simulink model "Demo_Shore"  (R2014a)
settings: Solver=FixedStepDiscrete  SolverMode=SingleTasking  StartTime=0.0  StopTime=inf  FixedStep=0.01  RelTol=1e-3
PostLoadFcn:
  | h_RPStest = RPStest;
model workspace (MAT data in the model file):
  gtest = 0
undefined symbols (not defined in the file or in its folder): avert, avert_gaze_dirs_chance, avert_gaze_duration_factor, avert_head_frequency_factor, avert_head_speed, BML, BML1, BML2, bmlsL, bmlsM, bodyBusyFlag, clock, emotion_amount_factor, faceBusyFlag, fileID, GAZE_WIN, gazing, mutual_gaze_duration_factor, P, pose_chanc_factor, pose_chance_factor, pose_change_flag, pose_frequency_factor, pose_lean, pose_lean_flag, pose_selfAdaptor_chance_factor, pose_speed, pr, serial, STATE_BEFORE, STATE_GO, STATE_OVER, STATE_READY, Stateflow
libraries: simulink x23, instrumentlib x6, lib_affectiveChar_behavior x3, realtime_pacer_lib x2, lib_affectiveChar_input x1
(part 5 of 7)

== stateflow chart Demo_Shore/CharacterControl/personalSpace_Controller ==
  state stateInit
    entry: gameState=14;
    TOO_CLOSE=1;TOO_FAR=2;NEUTRAL=0;
    farBuffer=0;closeBuffer=0;neutralBuffer=0;position=1;
    n=encStr2Arr(' ');bmlsM=[n n n n n];newBmlsM=[n n n n n];
    bmlsL=[n n n n n];newBmlsL=[n n n n n];
  note: Problem:
      | Sometimes locomotion BML is sent (visible in the vhmsgYarpRelais) but it is not running. Also smartbody shows duplicate msg id error. It seems that when too many BMLs are sent to smartbody some of them have same IDs.
  state wait
  note: if avert not 1
  state gazeSurprized
    entry: [P,BMLM]=walkInvadingTable(5) ;
    closeBuffer=closeBuffer+1;
    newBmlsM=insertQueue(bmlsM,BMLM);
    bmlsM=newBmlsM;
  state doIt3Times
    entry: position=2;
    closeBuffer=0;
  note: User is too close!
  state headNeuralGazeCamera
    entry: [P,BMLM]=walkInvadingTable(4) ;
    newBmlsM=insertQueue(bmlsM,BMLM);
    bmlsM=newBmlsM;
  state stateWalkBack
    entry:  [P,BMLM]=walkInvadingTable(2);
    newBmlsM=insertQueue(bmlsM,BMLM);  bmlsM=newBmlsM;
    closeBuffer=closeBuffer+1;
  state browUp
    entry: [P,BMLM]=walkInvadingTable(8) ;
    neutralBuffer=neutralBuffer+1;
    newBmlsM=insertQueue(bmlsM,BMLM);
    bmlsM=newBmlsM;
  state doIt3Times1
    entry: position=1;
    neutralBuffer=0;
  note: EXE ORDER IMPORTANT
  state checkUserCoord
  note: correct: [zChange==1]{position=0;}
  state idle
    entry: [P,BMLM]=walkInvadingTable(1);
    newBmlsM=insertQueue(bmlsM,BMLM);
    bmlsM=newBmlsM;
    neutralBuffer=neutralBuffer+1;
  note: User is in the middle!
  state wait2
  state leanFW
    entry: [P,BMLM]=walkInvadingTable(6) ;
    farBuffer=farBuffer+1;
    newBmlsM=insertQueue(bmlsM,BMLM);
    bmlsM=newBmlsM;
  state doIt3Times2
    entry: position=3;
    farBuffer=0;
  note: Problem:
      | We dont know where smatbody is standing (z pos). If smartbody does not run the locomotion BML sent for any reason (too many BMLs), we want to send locomodation BML again after a while to make sure the personal space is correct. On the other hand, we dont want the module to keep sending move bmls.
  state walkFW
    entry:  [P,BMLM]=walkInvadingTable(3) ;
    newBmlsM=insertQueue(bmlsM,BMLM);  bmlsM=newBmlsM;
    farBuffer=farBuffer+1;
  note: User is too far!
  state leanNeutral
    entry:  [P,BMLM]=walkInvadingTable(7) ;
    newBmlsM=insertQueue(bmlsM,BMLM); bmlsM=newBmlsM;
  (default) -> stateInit
  stateInit -> (junction 2)
  wait -> (junction 2)
  (junction 2) -> headNeuralGazeCamera [order 1] : [avert==1]
  (junction 2) -> checkUserCoord [order 2]
  idle -> wait [order 2] : after(5,secs)
  walkFW -> wait [order 2] : after(5,secs)
  stateWalkBack -> wait [order 2] : after(5,secs)
  doIt3Times1 -> wait : after(5,secs)
  doIt3Times2 -> wait : after(5,secs)
  doIt3Times -> wait : after(5,secs)
  checkUserCoord -> (junction 89) [order 3] : [[distance==TOO_CLOSE]&[position~=2]]
  (junction 89) -> gazeSurprized [order 2] : [closeBuffer<2]
  (junction 89) -> stateWalkBack [order 1] : [closeBuffer>=2]
  stateWalkBack -> doIt3Times [order 1] : [closeBuffer==5]
  gazeSurprized -> checkUserCoord
  headNeuralGazeCamera -> checkUserCoord
  checkUserCoord -> (junction 92) [order 2] : [[distance==NEUTRAL]&[position~=1]]
  (junction 92) -> browUp [order 1] : [neutralBuffer<2]
  wait2 -> checkUserCoord [order 1] : [zChange==1]{position=0;}
  idle -> doIt3Times1 [order 1] : [neutralBuffer==5]
  browUp -> checkUserCoord
  (junction 92) -> idle [order 2] : [neutralBuffer>=2]
  wait2 -> checkUserCoord [order 2] : [zChange~=1]
  checkUserCoord -> wait2 [order 4] : after(20,secs)
  checkUserCoord -> (junction 87) [order 1] : [[distance==TOO_FAR]&[position~=3]]
  leanFW -> checkUserCoord
  (junction 87) -> leanFW [order 2] : [farBuffer<2]
  walkFW -> doIt3Times2 [order 1] : [farBuffer==5]
  (junction 87) -> leanNeutral [order 1] : [farBuffer>=2]
  leanNeutral -> walkFW : after(2,secs)
  data: bmls function_input double size=[1000,5]; myBML function_input double size=[1000,1]; newBmls function_output double size=[1000,5]; p function_output double size=1; bmlID function_input double size=1; poseBML function_output double size=[1000,1]; bmls function_input double size=[1000,5]; myBML function_input double size=[1000,1]; newBmls function_output double size=[1000,5]; gameState output double size=1; STATE_READY data_store_memory size=1; STATE_OVER data_store_memory size=1; distance input double size=1; STATE_BEFORE data_store_memory size=1; BML1 data_store_memory size=[256,1]; P data_store_memory; pr data_store_memory; fileID data_store_memory; neutralBuffer local; closeBuffer local; NEUTRAL local; TOO_FAR local; TOO_CLOSE local; farBuffer local; zChange input; position local; avert data_store_memory; newBmlsM local double size=[1000,5]; bmlsM data_store_memory; BMLM local double size=[1000,1]; BMLL local double size=[1000,1]; newBmlsL local double size=[1000,5]; bmlsL data_store_memory; n local
  events: secs input RISING_EDGE_EVENT
  function newBmls =insertQueueLow(bmls,myBML):
    | function newBmls =insertQueueLow(bmls,myBML)
    |     full=1;
    |     t=encStr2Arr(' ');
    |     newBmls=[t t t t t];
    |     for i = 1:5
    |         if (isequal(bmls(:,i),t))
    |             %add to end of the queue where its empty
    |             bmls(:,i)=myBML;
    |             full=0;
    |             break
    |         end
    |     end
    |     if(full~=0)
    |             %if queue full, shift all elements to left which removes the first one, then add to end
    |             bmls(:,1)= bmls(:,2);
    |             bmls(:,2)= bmls(:,3);
    |             bmls(:,3)= bmls(:,4);
    |             bmls(:,5)=myBML;
    |     end
    |     newBmls=bmls;
  function [p,poseBML]=walkInvadingTable(bmlID):
    | function [p,poseBML]=walkInvadingTable(bmlID)
    | 
    | aVarTruthTableCondition_1 = false;
    | aVarTruthTableCondition_2 = false;
    | aVarTruthTableCondition_3 = false;
    | aVarTruthTableCondition_4 = false;
    | aVarTruthTableCondition_5 = false;
    | aVarTruthTableCondition_6 = false;
    | aVarTruthTableCondition_7 = false;
    | aVarTruthTableCondition_8 = false;
    | 
    | 
    | % n
    | 
    | aVarTruthTableCondition_1 = logical(bmlID==1);
    | 
    | % b
    | 
    | aVarTruthTableCondition_2 = logical(bmlID==2);
    | 
    | % f
    | 
    | aVarTruthTableCondition_3 = logical(bmlID==3);
    | 
    | % HN
    | 
    | aVarTruthTableCondition_4 = logical(bmlID==4);
    | 
    | % surprizeGaze
    | 
    | aVarTruthTableCondition_5 = logical(bmlID==5);
    | 
    | % leanFw
    | 
    | aVarTruthTableCondition_6 = logical(bmlID==6);
    | 
    | % leanNeutral
    | 
    | aVarTruthTableCondition_7 = logical(bmlID==7);
    | 
    | % browUp
    | 
    | aVarTruthTableCondition_8 = logical(bmlID==8);
    | 
    | if (aVarTruthTableCondition_1)
    |     aFcnTruthTableAction_1();
    | elseif (aVarTruthTableCondition_2)
    |     aFcnTruthTableAction_2();
    | elseif (aVarTruthTableCondition_3)
    |     aFcnTruthTableAction_3();
    | elseif (aVarTruthTableCondition_4)
    |     aFcnTruthTableAction_4();
    | elseif (aVarTruthTableCondition_5)
    |     aFcnTruthTableAction_5();
    | elseif (aVarTruthTableCondition_6)
    |     aFcnTruthTableAction_6();
    | elseif (aVarTruthTableCondition_7)
    |     aFcnTruthTableAction_7();
    | elseif (aVarTruthTableCondition_8)
    |     aFcnTruthTableAction_8();
    | else % Default
    |     aFcnTruthTableAction_1();
    | end
    | 
    | function aFcnTruthTableAction_1()
    | 
    | % Neutral
    | 
    | poseBML=encStr2Arr( '<?xml version="1.0" ?><act><bml><locomotion manner="walk" facing="gazeTarget"  sbm:accel="0.5" sbm:scootaccel="50" target="0 0"/></bml></act>');p=1;
    | 
    | function aFcnTruthTableAction_2()
    | 
    | % Back
    | 
    | poseBML=encStr2Arr( '<?xml version="1.0" ?><act><bml><locomotion manner="walk"  sbm:accel="0.5" sbm:scootaccel="50" facing="gazeTarget" target="0 -0.6"/></bml></act>');p=1;
    | 
    | function aFcnTruthTableAction_3()
    | 
    | % Forward
    | 
    | poseBML=encStr2Arr( '<?xml version="1.0" ?><act><bml><locomotion manner="walk" facing="gazeTarget"  sbm:accel="0.5" sbm:scootaccel="50" target="0 0.6"/></bml></act>');p=1;
    | 
    | function aFcnTruthTableAction_4()
    | 
    | % NeutralHead
    | 
    | poseBML=encStr2Arr('<?xml version="1.0" ?><act><bml><gaze target="gazeTarget" sbm:joint-range="EYES NECK" sbm:time-hint="1.5"/></bml></act>');p=1;
    | 
    | function aFcnTruthTableAction_5()
    | 
    | % surprisedGaze
    | 
    | poseBML=encStr2Arr('<?xml version="1.0" ?><act><bml><face type="FACS" start="0" end="5" side="BOTH" au="5" relax="3" amount="0.5"/><face type="FACS" start="0" end="5" side="BOTH" au="2" relax="3" amount="0.5"/></bml></act>');p=1;
    | 
    | function aFcnTruthTableAction_6()
    | 
    | % leanFW
    | 
    | poseBML=encStr2Arr('<?xml version="1.0" ?><act><bml><gaze angle="5" direction="DOWN" sbm:joint-range="HEAD BACK" sbm:time-hint="2" target="gazeTarget"/></bml></act>');p=1;
    | 
    | function aFcnTruthTableAction_7()
    | 
    | % leanNeutral
    | 
    | poseBML=encStr2Arr('<?xml version="1.0" ?><act><bml><gaze sbm:time-hint="2" target="gazeTarget"/></bml></act>');p=1;
    | 
    | function aFcnTruthTableAction_8()
    | 
    | % browUp
    | 
    | poseBML=encStr2Arr('<?xml version="1.0" ?><act><bml><face au="2" end="5" ready="1" relax="4" side="BOTH" start="0" stroke="3" type="facs"/></bml></act>');p=1;
  function newBmls =insertQueue(bmls,myBML):
    | function newBmls =insertQueue(bmls,myBML)
    |     full=1;
    |     t=encStr2Arr(' ');
    |     newBmls=[t t t t t];
    |     for i = 1:5
    |         if (isequal(bmls(:,i),t))
    |             %add to end of the queue where its empty
    |             bmls(:,i)=myBML;
    |             full=0;
    |             break
    |         end
    |     end
    |     if(full~=0)
    |             %if queue full, shift all elements to left which removes the first one, then add to end
    |             bmls(:,1)= bmls(:,2);
    |             bmls(:,2)= bmls(:,3);
    |             bmls(:,3)= bmls(:,4);
    |             bmls(:,5)=myBML;
    |     end
    |     newBmls=bmls;
